simulink model "FSM_modelC"  (R2021a)
settings: Solver=VariableStepAuto  StartTime=0.0  StopTime=10.0  RelTol=1e-3
settings Model: Creator=ASWADH  LastModifiedBy=lenovo
settings DebuggingCC: SignalRangeChecking=warning  UnderSpecifiedDimensionMsg=warning

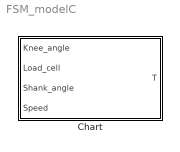
== system FSM_modelC ==
  Chart : Stateflow chart  TreatAsAtomicUnit=on

== stateflow chart FSM_modelC/Chart ==
  state WALKINGSPEED2
    state Upon_Swing
      entry:USwing_Torque
      during : disp(T)
    state Swing_Flexion
      entry:SFlexion_torque
      during : disp(T)
    state Stance
      entry:Stance_torque
      during : disp(T)
    state Upon_Stance
      entry:UStance_Torque
      during : disp(T)
    state SwingExtension
      entry:SExtension_Torque
      during : disp(T)
    (default) -> Stance
    Upon_Swing -> Swing_Flexion : [Knee_angle > 0, Shank_angle < 0, Load_cell == 0]
    Stance -> Upon_Swing : [Knee_angle > 0,Shank_angle == 0,Load_cell == 0]
    Upon_Stance -> Stance : [Knee_angle == 0,Shank_angle == 0,Load_cell == 1]
    Swing_Flexion -> SwingExtension : [Knee_angle < 0,Shank_angle > 0,Load_cell == 0]
    SwingExtension -> Upon_Stance : [Knee_angle == 0, Shank_angle > 0,Load_cell == 1]
  state GAITSPEED
  GAITSPEED -> WALKINGSPEED2 : [Speed <= 2]
  (default) -> GAITSPEED
  data: Knee_angle input; Load_cell input; Shank_angle input; Speed input; T output
  function USwing_Torque:
    | function USwing_Torque
    |  knee_angle = int32(30);
    |  Leg_angle =  int32(0);
    | % Connect to the IMU sensor using the serial interface
    | % Read the knee angle data from the IMU sensor
    | knee_angle = load('knee_angle_data.mat');
    | 
    | %computation for Leg_angle
    | leg_angle = acos((sin(knee_angle)/l_shank*l_leg));
    | 
    | % Calculate the time step
    | time_step = 0.01;
    | 
    | %at Swing phase (on set of swing phase)
    | % Calculate the rate of change of the leg angle using finite difference method
    | d_leg_angle = diff(Leg_angle) / time_step;
    | 
    | % Evaluate the appropriate function based on the limits
    | if d_leg_angle > 0
    | T = T1 ;
    | elseif d_leg_angle < 0
    | T = T2 ;
    | end 
    |  % flexion gain calculation % Load the EMG and knee angle data
    | emg_data = load('emg_data.mat');
    | knee_angle_data = load('knee_angle_data.mat');
    | 
    | % Filter the EMG data to remove high-frequency noise
    | filtered_emg = highpass(emg_data, 20, 1000);
    | 
    | % Normalize the EMG data to a standard range
    | normalized_emg = (filtered_emg - min(filtered_emg)) / (max(filtered_emg) - min(filtered_emg));
    | 
    | % Determine the muscle activation onset
    | threshold = 0.5;
    | activation_onset = find(normalized_emg >= threshold, 1);
    | 
    | % Calculate the muscle length change
    | muscle_length_start = calculate_muscle_length(knee_angle_data(1));
    | muscle_length_end = calculate_muscle_length(knee_angle_data(activation_onset));
    | muscle_length_change = muscle_length_end - muscle_length_start;
    | 
    | % Calculate the knee angle change
    | knee_angle_change = knee_angle_data(activation_onset) - knee_angle_data(1);
    | 
    | % Calculate the flexion gain
    | Flexion_gain = muscle_length_change / knee_angle_change;
    | 
    | % Display the result
    | disp(['Flexion_gain: ', num2str(Flexion_gain)])
    |  
    | %at Swing phase (on set of swing phase)
    | T1 = 0;
    | T2 = Flexion_gain*Leg_angle;
    |  
    | % Display the Result
    | disp(T)
  function SFlexion_torque:
    | function SFlexion_torque
    | 
    | % define the knee angle in degrees
    | knee_angle_deg = 30;
    | % convert the knee angle to radians
    | knee_angle_rad = deg2rad(knee_angle_deg);
    | % Connect to the IMU sensor using the serial interface
    | % Read the knee angle data from the IMU sensor
    | knee_angle = load('knee_angle_data.mat');
    | l_shank = 0.400; % example value for the shank length
    | l_leg = 0.950; % example value for the leg length
    | leg_angle = acos((sin(knee_angle_rad))/(l_shank*l_leg));
    | 
    | % Calculate the time step
    | time_step = 0.01;
    | 
    | %at Swing phase (on set of swing phase)
    | % Calculate the rate of change of the leg angle using finite difference method
    | d_leg_angle = diff(leg_angle) / time_step;
    | 
    | % Target leg angle 
    | Tgt_legangle = 30;%subject to change
    | 
    | % Calculate the time step
    | time_step = 0.01;
    | 
    | % At Swing phase Flexion (on set of swing phase flexion)
    | % Calculate the rate of change of the leg angle using finite difference method
    | d_leg_angle = diff(leg_angle) / time_step;
    | 
    | % Calculate the rate of change of the knee angle using finite difference method
    | d_knee_angle = diff(knee_angle_deg) / time_step;
    | 
    | % Flexion gain calculation
    | % Load the EMG and knee angle data
    | emg_data = load('emg_data.mat');
    | knee_angle_data = load('knee_angle_data.mat');
    | 
    | % Filter the EMG data to remove high-frequency noise
    | filtered_emg = highpass(emg_data, 20, 1000);
    | 
    | % Normalize the EMG data to a standard range
    | normalized_emg = (filtered_emg - min(filtered_emg)) / (max(filtered_emg) - min(filtered_emg));
    | 
    | % Determine the muscle activation onset
    | threshold = 0.5;
    | activation_onset = find(normalized_emg >= threshold, 1);
    | 
    | % Calculate the muscle length change
    | muscle_length_start = 0; % Replace with an appropriate value or function
    | muscle_length_end = 0; % Replace with an appropriate value or function
    | muscle_length_change = muscle_length_end - muscle_length_start;
    | 
    | % Calculate the knee angle change
    | d_knee_angle = knee_angle_data(activation_onset) - knee_angle_data(1);
    | 
    | % Calculate the flexion gain
    | Flexion_gain = muscle_length_change / d_knee_angle;
    | 
    | % Display the result
    | disp(['Flexion_gain: ', num2str(Flexion_gain)])
    | 
    | % Evaluation of functions based on limits
    | if d_knee_angle >= 0
    |     T = T1;
    | elseif ((d_knee_angle) < 0 && knee_angle < leg_angle)
    |     T = T2;
    | else
    |     T = 0;
    | end
    | 
    | % Torque computation
    | T1 = (-Flexion_gain*knee_angle);
    | T2 = ((-Flexion_gain*knee_angle)*(Leg_angle - Tgt_legangle)*(d_leg_angle-d_knee_angle));
    | 
    | disp(T);
  function Stance_torque:
    | function Stance_torque
    |  F_Muscletendon = 24610.07981; 
    |  Variablemoment = -261.9647304; 
    |  T = F_Muscletendon*Variablemoment;
    | disp(T)
  function UStance_Torque:
    | function UStance_Torque
    |  GRF = 65;
    |  F_Muscletendon = 24610.07981; 
    |  Variablemoment = -261.9647304; 
    |  T0 = F_Muscletendon*Variablemoment;
    |  T = T0*GRF + (SwingTorque*(1-GRF));
    |  disp(T);
  function SExtension_Torque:
    | function SExtension_Torque
    |  knee_angle = int32(30);
    |  Leg_angle =  int32(0);
    |  % Read the knee angle data from the IMU sensor
    | knee_angle = load('knee_angle_data.mat');
    | %computation for Leg_angle
    | leg_angle = acos((sin(knee_angle)/l_shank*l_leg));
    | 
    | % Calculate the time step
    | time_step = 0.01;
    | 
    | %at Swing phase Extension(swing phase extension)
    | % Calculate the rate of change of the leg angle using finite difference method
    | d_leg_angle = diff(Leg_angle) / time_step;
    | 
    | % flexion gain calculation % Load the EMG and knee angle data
    | emg_data = load('emg_data.mat');
    | knee_angle_data = load('knee_angle_data.mat');
    | 
    | % Filter the EMG data to remove high-frequency noise
    | filtered_emg = highpass(emg_data, 20, 1000);
    | 
    | % Normalize the EMG data to a standard range
    | normalized_emg = (filtered_emg - min(filtered_emg)) / (max(filtered_emg) - min(filtered_emg));
    | 
    | % Determine the muscle activation onset
    | threshold = 0.5;
    | activation_onset = find(normalized_emg >= threshold, 1);
    | 
    | % Calculate the muscle length change
    | muscle_length_start = calculate_muscle_length(knee_angle_data(1));
    | muscle_length_end = calculate_muscle_length(knee_angle_data(activation_onset));
    | muscle_length_change = muscle_length_end - muscle_length_start;
    | 
    | % Calculate the knee angle change
    | knee_angle_change = knee_angle_data(activation_onset) - knee_angle_data(1);
    | 
    | % Calculate the flexion gain
    | Flexion_gain = muscle_length_change / knee_angle_change;
    | 
    | % Display the result
    | disp(['Flexion_gain: ', num2str(Flexion_gain)]);
    | 
    | % Evaluate the approriate function based on limits
    | Legangle_Threshold = 0.5;% variable 
    | Max_Kneeretraction_velocity = 150 ; %(basically differs between 150 - 200)
    | if leg_angle < Legangle_Threshold
    |     T = T1;
    | elseif d_leg_angle < Max_Kneeretraction_velocity
    |     T = 0;
    | end 
    |  T1 =  Flexion_gain(Legangle_Threshold - leg_angle)*(1 - (d_leg_angle/Max_Kneeretraction_velocity));
    |  disp(T)
